simulink model "SIM_4_TANK"  (R2023b)
settings: Solver=VariableStepAuto  StartTime=0.0  StopTime=1200  RelTol=1e-3
values from neighbouring files (symbols this model uses):
  Ts = 3    [MHE_compute.m]    (also in sample_time.m)
libraries: simulink x1
settings Model: Creator=akeebismail  LastModifiedBy=akeebismail

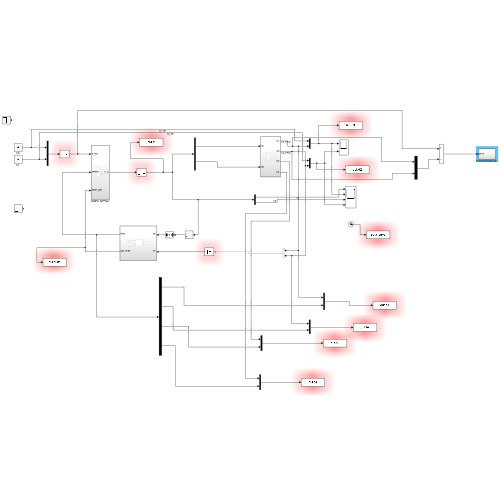
[thumbnail: Simulink's stored preview of the top-level diagram]
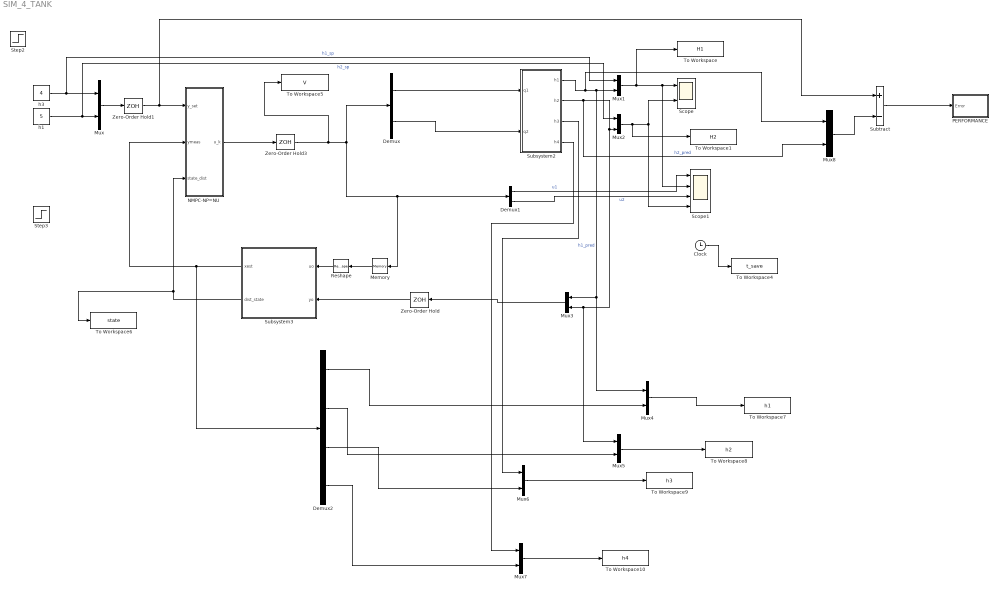
== system SIM_4_TANK ==
  Clock : Clock
  Demux : Demux  Outputs=2
  Demux1 : Demux  Outputs=2
  Demux2 : Demux
  Memory : Memory  InitialCondition=[55;75]
  Mux{,1..8} (9 alike) : Mux  Inputs=2
  NMPC-NP=NU : Subsystem
  PERFORMANCE : Subsystem
  Reshape : Reshape  OutputDimensionality=Row vector (2-D)
  Scope : Scope  NumInputPorts=2
  Scope1 : Scope  NumInputPorts=4
  Step2 : Step  Time=500  Before=4  After=3.9  SampleTime=0
  Step3 : Step  Time=500  Before=5  After=6.5  SampleTime=0
  Subsystem2 : Subsystem
  Subsystem3 : Subsystem
  Subtract : Sum  Inputs=+-
  To Workspace : ToWorkspace  VariableName=H1  SaveFormat=Timeseries  SampleTime=Ts
  To Workspace1 : ToWorkspace  VariableName=H2  SaveFormat=Timeseries  SampleTime=Ts
  To Workspace10 : ToWorkspace  VariableName=h4  SaveFormat=Timeseries  SampleTime=Ts
  To Workspace4 : ToWorkspace  VariableName=t_save  SaveFormat=Timeseries  SampleTime=Ts
  To Workspace5 : ToWorkspace  VariableName=V  SaveFormat=Timeseries  SampleTime=Ts
  To Workspace6 : ToWorkspace  VariableName=state  SaveFormat=Timeseries  SampleTime=Ts
  To Workspace7 : ToWorkspace  VariableName=h1  SaveFormat=Timeseries  SampleTime=Ts
  To Workspace8 : ToWorkspace  VariableName=h2  SaveFormat=Timeseries  SampleTime=Ts
  To Workspace9 : ToWorkspace  VariableName=h3  SaveFormat=Timeseries  SampleTime=Ts
  Zero-Order Hold : ZeroOrderHold  SampleTime=Ts
  Zero-Order Hold1 : ZeroOrderHold  SampleTime=Ts
  Zero-Order Hold3 : ZeroOrderHold  SampleTime=Ts
  h1 : Constant  Value=5
  h3 : Constant  Value=4
  wires:
  Mux/1 -> Zero-Order Hold1/1
  NMPC-NP=NU/1(u_k) -> Zero-Order Hold3/1
  h3/1 -> Mux/1, Mux1/1  "h1_sp"
  Demux1/1 -> Scope1/1  "u1"
  Demux/2 -> Subsystem2/2(q2)
  Demux1/2 -> Scope1/3  "u2"
  Mux1/1 -> To Workspace/1, Scope1/2, Scope/1
  Subsystem2/1(h1) -> Mux8/1, Mux4/1, Mux3/1, Mux1/2  "h1_pred"
  Subsystem2/2(h2) -> Mux8/2, Mux5/1, Mux3/2, Mux2/2  "h2_pred"
  Zero-Order Hold/1 -> Subsystem3/2(yo)
  h1/1 -> Mux/2, Mux2/1  "h2_sp"
  Mux3/1 -> Zero-Order Hold/1
  Mux2/1 -> To Workspace1/1, Scope1/4, Scope/2
  Memory/1 -> Reshape/1
  Reshape/1 -> Subsystem3/1(uo)
  Demux/1 -> Subsystem2/1(q1)
  Subsystem3/2(dist_state) -> To Workspace6/1, NMPC-NP=NU/3(state_dist)
  Zero-Order Hold1/1 -> Subtract/1, NMPC-NP=NU/1(y_set)
  Zero-Order Hold3/1 -> To Workspace5/1, Demux/1, Memory/1, Demux1/1
  Subsystem3/1(xest) -> Demux2/1, NMPC-NP=NU/2(ymeas)
  Subsystem2/3(h3) -> Mux6/1
  Subsystem2/4(h4) -> Mux7/1
  Clock/1 -> To Workspace4/1
  Demux2/1 -> Mux4/2
  Demux2/2 -> Mux5/2
  Demux2/3 -> Mux6/2
  Demux2/4 -> Mux7/2
  Mux4/1 -> To Workspace7/1
  Mux5/1 -> To Workspace8/1
  Mux6/1 -> To Workspace9/1
  Mux7/1 -> To Workspace10/1
  Mux8/1 -> Subtract/2
  Subtract/1 -> PERFORMANCE/1(Error)

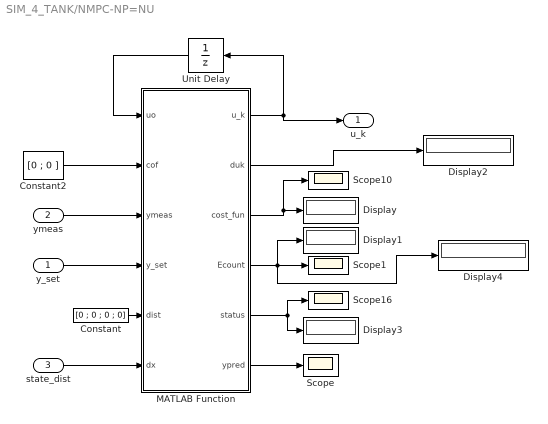
== system SIM_4_TANK/NMPC-NP=NU ==
  y_set : Inport
  ymeas : Inport  Port=2
  state_dist : Inport  Port=3
  Constant : Constant  Value=[0 ; 0 ; 0 ; 0]
  Constant2 : Constant  Value=[0 ; 0 ]
  Display{,1..4} (5 alike) : Display
  MATLAB Function : MATLAB Function  TreatAsAtomicUnit=on
  Scope{,1,10,16} (4 alike) : Scope
  Unit Delay : UnitDelay  InitialCondition=[55;75]  SampleTime=Ts  HasFrameUpgradeWarning=on
  u_k : Outport  VectorParamsAs1DForOutWhenUnconnected=off
  wires:
  Unit Delay/1 -> MATLAB Function/1(uo)
  MATLAB Function/6(ypred) -> Scope/1
  MATLAB Function/4(Ecount) -> Display4/1, Display1/1, Scope1/1
  MATLAB Function/5(status) -> Scope16/1, Display3/1
  MATLAB Function/1(u_k) -> u_k/1, Unit Delay/1
  MATLAB Function/3(cost_fun) -> Scope10/1, Display/1
  Constant2/1 -> MATLAB Function/2(cof)
  ymeas/1 -> MATLAB Function/3(ymeas)
  y_set/1 -> MATLAB Function/4(y_set)
  MATLAB Function/2(duk) -> Display2/1
  Constant/1 -> MATLAB Function/5(dist)
  state_dist/1 -> MATLAB Function/6(dx)

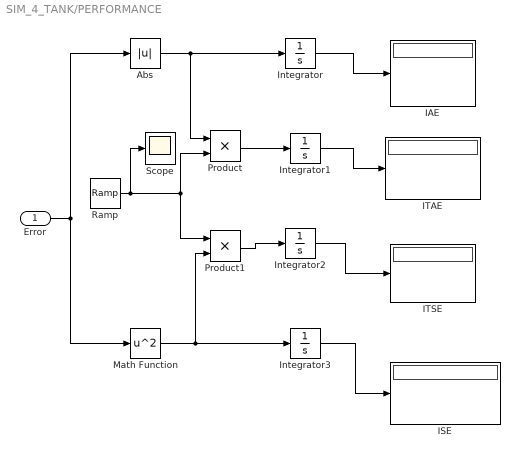
== system SIM_4_TANK/PERFORMANCE ==
  Error : Inport
  Abs : Abs  SaturateOnIntegerOverflow=off
  IAE : Display
  ISE : Display
  ITAE : Display
  ITSE : Display
  Integrator{,1..3} (4 alike) : Integrator
  Math Function : Math  Operator=square  SignedPower=on
  Product : Product  RndMeth=Zero
  Product1 : Product  RndMeth=Zero
  Ramp : simulink/Sources/Ramp  slope=1  start=0  InitialOutput=0
  Scope : Scope
  wires:
  Error/1 -> Math Function/1, Abs/1
  Abs/1 -> Integrator/1, Product/1
  Integrator/1 -> IAE/1
  Ramp/1 -> Product/2, Product1/1, Scope/1
  Math Function/1 -> Integrator3/1, Product1/2
  Product1/1 -> Integrator2/1
  Product/1 -> Integrator1/1
  Integrator3/1 -> ISE/1
  Integrator2/1 -> ITSE/1
  Integrator1/1 -> ITAE/1

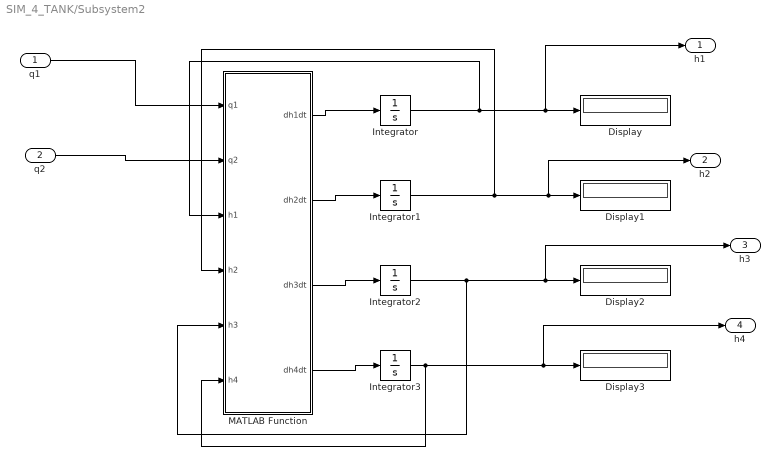
== system SIM_4_TANK/Subsystem2 ==
  q1 : Inport
  q2 : Inport  Port=2
  Display{,1..3} (4 alike) : Display
  Integrator{,1..3} (4 alike) : Integrator
  MATLAB Function : MATLAB Function  TreatAsAtomicUnit=on
  h1 : Outport
  h2 : Outport  Port=2
  h3 : Outport  Port=3
  h4 : Outport  Port=4
  wires:
  Integrator1/1 -> MATLAB Function/4(h2), h2/1, Display1/1
  q2/1 -> MATLAB Function/2(q2)
  Integrator3/1 -> MATLAB Function/6(h4), h4/1, Display3/1
  q1/1 -> MATLAB Function/1(q1)
  Integrator2/1 -> MATLAB Function/5(h3), h3/1, Display2/1
  MATLAB Function/2(dh2dt) -> Integrator1/1
  MATLAB Function/1(dh1dt) -> Integrator/1
  MATLAB Function/4(dh4dt) -> Integrator3/1
  MATLAB Function/3(dh3dt) -> Integrator2/1
  Integrator/1 -> MATLAB Function/3(h1), h1/1, Display/1

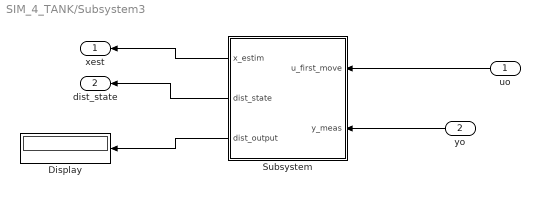
== system SIM_4_TANK/Subsystem3 ==
  uo : Inport
  yo : Inport  Port=2
  Display : Display
  Subsystem : Subsystem
  xest : Outport
  dist_state : Outport  Port=2
  wires:
  Subsystem/1(x_estim) -> xest/1
  Subsystem/2(dist_state) -> dist_state/1
  Subsystem/3(dist_output) -> Display/1
  uo/1 -> Subsystem/1(u_first_move)
  yo/1 -> Subsystem/2(y_meas)

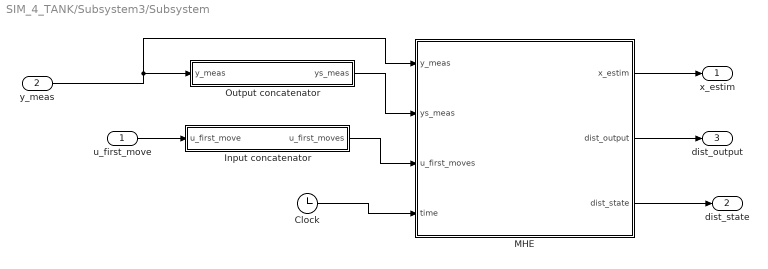
== system SIM_4_TANK/Subsystem3/Subsystem ==
  u_first_move : Inport  PortDimensions=[1,2]
  y_meas : Inport  Port=2  PortDimensions=[1,2]
  Clock : Clock
      settings: Decimation=20
  Input concatenator : Subsystem
  MHE : MATLAB Function  TreatAsAtomicUnit=on
  Output concatenator : Subsystem
  x_estim : Outport
  dist_state : Outport  Port=2
  dist_output : Outport  Port=3
  wires:
  Input concatenator/1(u_first_moves) -> MHE/3(u_first_moves)
  MHE/3(dist_state) -> dist_state/1
  MHE/2(dist_output) -> dist_output/1
  Clock/1 -> MHE/4(time)
  u_first_move/1 -> Input concatenator/1(u_first_move)
  MHE/1(x_estim) -> x_estim/1
  y_meas/1 -> Output concatenator/1(y_meas), MHE/1(y_meas)
  Output concatenator/1(ys_meas) -> MHE/2(ys_meas)

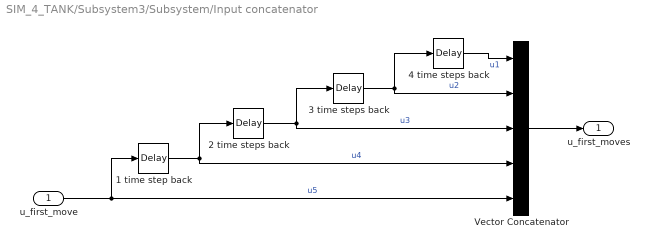
== system SIM_4_TANK/Subsystem3/Subsystem/Input concatenator ==
  u_first_move : Inport
  1 time step back : TransportDelay  DelayTime=3  InitialOutput=[55,75]
  2 time steps back : TransportDelay  DelayTime=3  InitialOutput=[55,75]
  3 time steps back : TransportDelay  DelayTime=3  InitialOutput=[55,75]
  4 time steps back : TransportDelay  DelayTime=3  InitialOutput=[55,75]
  Vector Concatenator : Concatenate  NumInputs=5  Mode=Multidimensional array
  u_first_moves : Outport  PortDimensions=[5,2]  VectorParamsAs1DForOutWhenUnconnected=off
  wires:
  Vector Concatenator/1 -> u_first_moves/1
  u_first_move/1 -> 1 time step back/1, Vector Concatenator/5  "u5"
  4 time steps back/1 -> Vector Concatenator/1  "u1"
  3 time steps back/1 -> 4 time steps back/1, Vector Concatenator/2  "u2"
  2 time steps back/1 -> 3 time steps back/1, Vector Concatenator/3  "u3"
  1 time step back/1 -> 2 time steps back/1, Vector Concatenator/4  "u4"

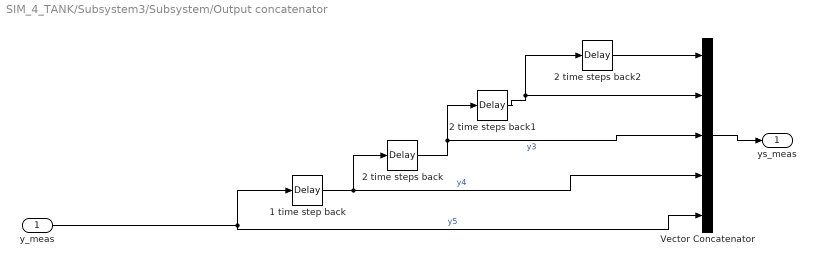
== system SIM_4_TANK/Subsystem3/Subsystem/Output concatenator ==
  y_meas : Inport
  1 time step back : TransportDelay  DelayTime=3  InitialOutput=[4,5]
  2 time steps back : TransportDelay  DelayTime=3  InitialOutput=[4,5]
  2 time steps back1 : TransportDelay  DelayTime=3  InitialOutput=[4,5]
  2 time steps back2 : TransportDelay  DelayTime=3  InitialOutput=[4,5]
  Vector Concatenator : Concatenate  NumInputs=5  Mode=Multidimensional array
  ys_meas : Outport  PortDimensions=[5,2]  VectorParamsAs1DForOutWhenUnconnected=off
  wires:
  2 time steps back2/1 -> Vector Concatenator/1
  2 time steps back1/1 -> Vector Concatenator/2, 2 time steps back2/1
  Vector Concatenator/1 -> ys_meas/1
  2 time steps back/1 -> Vector Concatenator/3, 2 time steps back1/1  "y3"
  1 time step back/1 -> 2 time steps back/1, Vector Concatenator/4  "y4"
  y_meas/1 -> 1 time step back/1, Vector Concatenator/5  "y5"

== matlab function SIM_4_TANK/NMPC-NP=NU/MATLAB Function ==
  data: uo input size=[2,1]; cof input; ymeas input; u_k output size=[2,1]; duk output; y_set input size=[2,1]; dist input size=[4,1]; cost_fun output size=1; Ecount output; status output; ypred output; dx input
function [u_k,duk,cost_fun,Ecount,status,ypred] = NMPC_FT(uo,cof,ymeas,y_set,dist,dx)

%#codegen
coder.extrinsic('ucompute')

r1=y_set(1)  ; 
r2=y_set(2)  ; 

xo=ymeas  ;


d1 = dist(1,:);
d2 = dist(2,:);
d3 = dist(3,:);
d4 = dist(4,:);

%MPC TUNNING PARAMETERS
Np=10;  % 3  %   10  60  40
%Nu=1;   %  2   %  1


%%%%%%%%%%%%%%%%%%%%%%%%%%%%%%%%%%%%%%%%%%%%%%%%%%%%%%%%%%%%%

% WEIGHTS ON Y, U AND DELTA_U

dTs=3 ;
Wy1=1  ;    Wy2=1;      
Wu1=0.5 ;      Wu2=0.5;        
 Wdu1=10;    Wdu2=10;     
%Wdu1=0.1;    Wdu2=0.1;  



% TERMINAL CONDITIONS


% SAMPLING TIME FOR DISCRETIZATION
hstep=0.1; %sampling time of 10 is with less interation while 5 is smoother but higher interaction
Nsteps=2 ;% Nsteps=10 ; % Nsteps=20 ;
%h=0.001;

%%%%%%%%%%%%%%%%%%%%%%%%%%
% PROCESS CONSTRAINTS ON Y, U AND DELTA_U
x1min=0;  x2min=0; 
x1max=32; x2max=32;

u1min=15;   u2min=10; 
u1max=150;   u2max=98;   



du1min=-10 ; du2min=-10;  
du1max=10 ;  du2max=10 ;  



DUMIN_colvector=[du1min*ones(Np,1) ; du2min*ones(Np,1) ];
DUMAX_colvector=[du1max*ones(Np,1) ; du2max*ones(Np,1) ];


%%%%%%%%%%%%%%%%%%%%%%%%%%%%%%%%%%%%%%%%%%%%%%%
%CURRENT PROCESS STATES AND INPUTS

%[sys, xp, order] = Cascaded_tank_model([],[],[],'sizes') ;
%xo=xp  ;     
%xo=[14.29 ; 13.51 ; 16.06];
%uo=[100 ; 0.4 ; 0.2];

% STARTING POINT FOR THE OPTIMIZATION ALGORITHM
n0=[0.1;0.1];
U_initial=[n0(1)*ones(Np,1) ;  n0(2)*ones(Np,1)];
% U_initial=[0.01*ones(Nu,1);0.01*ones(Nu,1);0.01*ones(Nu,1)];

% PROCESS INPUT TRAJECTORY

u1set=55;
u2set=75;

%%%%%%%%%%%%%%%%%%%%%%%%

fcost=inf  ;
u_first_move=[0;0]  ;
ypred=[0;0]  ;
Ecount=0  ;
exitflag=2;


[u_first_move,fcost,Ecount,exitflag,ypred]=ucompute(r1,r2,u1set,u2set,Wy1,Wy2...
         ,Wu1,Wu2,Wdu1,Wdu2,xo,uo,hstep,Nsteps,Np,d1,d2,d3,d4,cof,dx...
         ,x1min,x2min,x1max,x2max,u1min,u2min,u1max,u2max...
          ,du1min, du2min, du1max, du2max...
         ,U_initial,DUMIN_colvector,DUMAX_colvector)  ;
     
duk = u_first_move ;     

u_k=uo + u_first_move  ;
%u_k=uo ;


status = exitflag;
cost_fun=fcost  ;

== matlab function SIM_4_TANK/Subsystem2/MATLAB Function ==
  data: q1 input; dh1dt output; q2 input; h1 input; h2 input; h3 input; h4 input; dh2dt output; dh3dt output; dh4dt output
function [dh1dt,dh2dt,dh3dt,dh4dt] = fcn(q1,q2,h1,h2,h3,h4)
values = {0.97,0.42,0.74,0.426,0.8542,0.7126,0.7722,0.5149,35,35,39,39,981,0.23,0.19};
[a1,a3,a2,a4,alpha1,alpha3,alpha2,alpha4,A1,A3,A2,A4,g,gamma1,gamma2] = values{:};

%F = k1 * v1;
%F2 = k2 * v2;

    dh1dt = -(a1*alpha1/A1) * sqrt(2 * g * h1) + (a3*alpha3/A1) * sqrt(2 * g * h3) + (gamma1 * q1) / A1;
    dh2dt = -(a2*alpha2/A2) * sqrt(2 * g * h2) + (a4*alpha4/A2) * sqrt(2 * g * h4) + (gamma2 * q2) / A2;
    dh3dt = -(a3*alpha3/A3) * sqrt(2 * g * h3) + ((1 - gamma2) * q2) / A3;
    dh4dt = -(a4*alpha4/A4) * sqrt(2 * g * h4) + ((1 - gamma1) * q1) / A4;

end

== matlab function SIM_4_TANK/Subsystem3/Subsystem/MHE ==
  data: y_meas input; ys_meas input; x_estim output; u_first_moves input; time input; dist_output output; dist_state output
function [x_estim,dist_output,dist_state] = MHE_4_tanks(y_meas,ys_meas,u_first_moves,time)

coder.extrinsic('MHE_compute','clear_var');

N_MHE=5  ;
% Ts=2 ;


if time < 15
    
    x_estim =  [0;0;0;0]  ;
   % x_estim = [17;17;17];
    %x_estim = [5.898;1.8];
    dist_output = [0;0];
    dist_state = [0;0;0;0];
    clear_var();
else
    
    [x_estim,dist_state,dist_output] = MHE_compute(ys_meas,u_first_moves,N_MHE,y_meas);
    %Note that our horizon must be constant here. It is chosen as 5.
end

end
